simulink model "Establecimiento"  (R2023b)
settings: Solver=VariableStepAuto  StartTime=0.0  StopTime=0.05  RelTol=1e-3
undefined symbols (not defined in the file): id0, L_d, R_s_actual, R_sREF
settings Model: Creator=tomas  LastModifiedBy=tomas

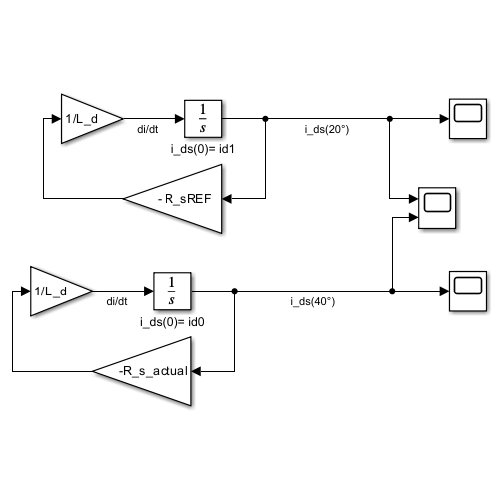
[thumbnail: Simulink's stored preview of the top-level diagram]
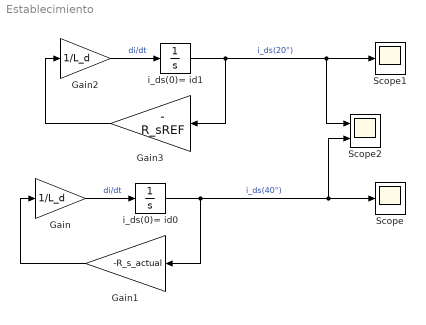
== system Establecimiento ==
  Gain : Gain  Gain=1/L_d
  Gain1 : Gain  Gain=-R_s_actual
  Gain2 : Gain  Gain=1/L_d
  Gain3 : Gain  Gain=- R_sREF
  Scope : Scope
  Scope1 : Scope
  Scope2 : Scope  NumInputPorts=2
  i_ds(0)= id0 : Integrator  InitialCondition=id0
  i_ds(0)= id1 : Integrator  InitialCondition=id0
  wires:
  i_ds(0)= id0/1 -> Gain1/1, Scope2/2, Scope/1  "i_ds(40°)"
  Gain1/1 -> Gain/1
  Gain/1 -> i_ds(0)= id0/1  "di/dt"
  Gain3/1 -> Gain2/1
  Gain2/1 -> i_ds(0)= id1/1  "di/dt"
  i_ds(0)= id1/1 -> Scope1/1, Scope2/1, Gain3/1  "i_ds(20°)"
